simulink model "model"  (R2023b)
settings: Solver=VariableStepAuto  StartTime=0  StopTime=simtime  FixedStep=0.001  RelTol=1e-3
values from neighbouring files (symbols this model uses):
  A = 93.086154    [project1.m]
  Af = 2.2    [project1.m]
  B = 2.5373490    (= 2.537349)    [project1.m]
  C = 0.38382359    [project1.m]
  Cd = 0.3    [project1.m]
  Crr = 0.015    [project1.m]
  D = 0    [project1.m]
  g0 = 3.173    [project1.m]
  I = 0.1    [project1.m]
  M = 1200    [project1.m]
  P = 10    [project1.m]
  Rw = 0.281154    [project1.m]
libraries: autolibshared x1
settings Model: Creator=qwert  LastModifiedBy=chall2022

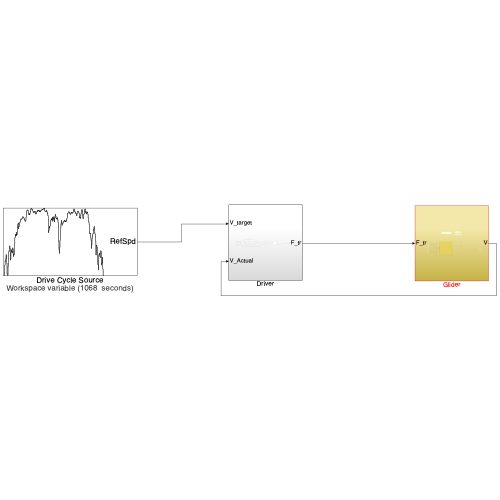
[thumbnail: Simulink's stored preview of the top-level diagram]
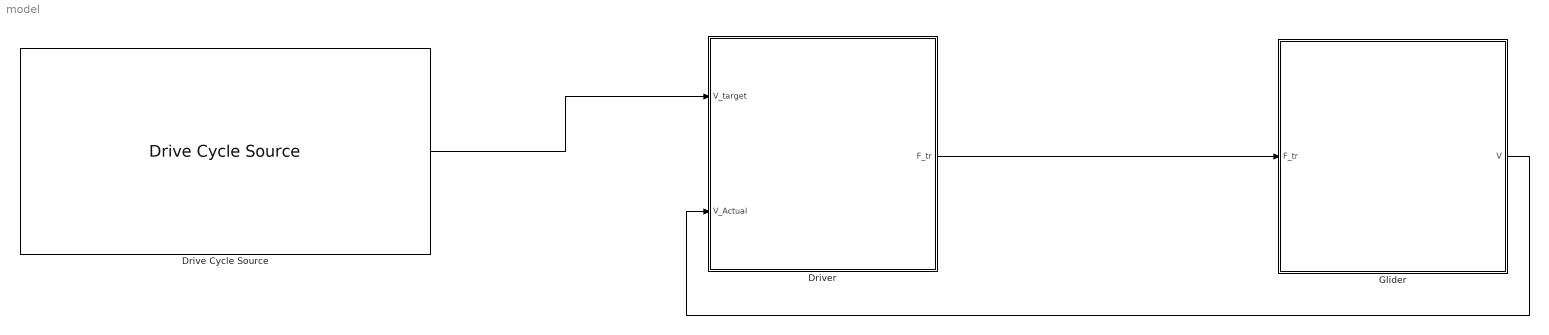
== system model ==
  Drive Cycle Source : autolibshared/Drive Cycle Source  cycleVar=Workspace variable  wsVar=Drivecycle  fileVar=cycleFTP75.mat  tfinal="1068  seconds"  cycleRepeat=off  outAccPort=off  outGearPort=off  gearList=No gear data  t_wot1=5  xdot_woto=0  xdot_wot1=30  t_wot2=20  xdot_wot2=0  t_wotend=30  srcUnit=m/s  outUnit=m/s  srcAccUnit=m/s/s  outAccUnit=m/s^2  dt=0  aMode=1  faultOption=off  velBnd=2  velBndUnit=mph  inUnit=m/s  timeBnd=1  failOption=off  stopSim=off  maxFaultCnt=10  maxFaultTime=2  maxTotFaultTime=15  traceOption=off  dtTrace=1  traceWindow=10  lastDCname=Custom Data Set  lastOutUnit=mph  lastDT=0  lastTB=1  lastSB=2  forceCalcBound=off
  Driver : Subsystem
  Glider : Subsystem
  wires:
  Driver/1(F_tr) -> Glider/1(F_tr)
  Drive Cycle Source/1 -> Driver/1(V_target)
  Glider/1(V) -> Driver/2(V_Actual)

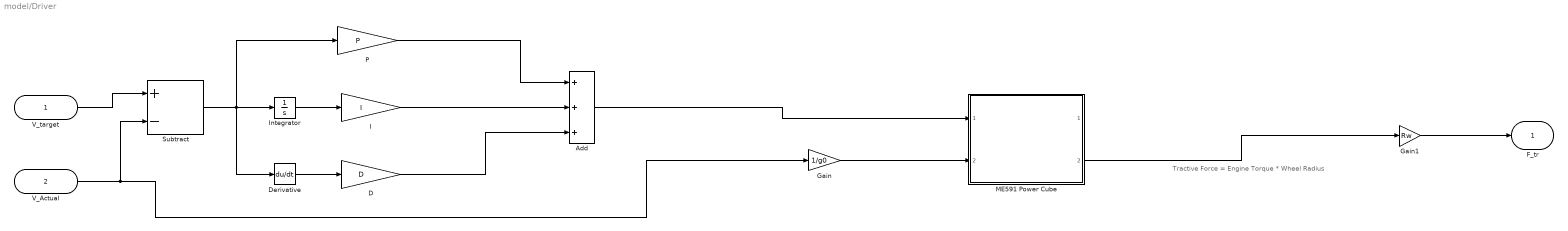
== system model/Driver ==
  note: Tractive Force = Engine Torque * Wheel Radius
  V_target : Inport
  V_Actual : Inport  Port=2
  Add : Sum  Inputs=+++
  D : Gain  Gain=D
  Derivative : Derivative
  Gain : Gain  Gain=1/g0
  Gain1 : Gain  Gain=Rw
  I : Gain  Gain=I
  Integrator : Integrator
  ME591 Power Cube : Subsystem  ReferencedSubsystem=ME591_Power_Cube
  P : Gain  Gain=P
  Subtract : Sum  Inputs=+-
  F_tr : Outport
  wires:
  I/1 -> Add/2
  P/1 -> Add/1
  D/1 -> Add/3
  Derivative/1 -> D/1
  Integrator/1 -> I/1
  V_Actual/1 -> Subtract/2, Gain/1
  Gain/1 -> ME591 Power Cube/2
  Gain1/1 -> F_tr/1
  Add/1 -> ME591 Power Cube/1
  V_target/1 -> Subtract/1
  Subtract/1 -> Derivative/1, P/1, Integrator/1
  ME591 Power Cube/2 -> Gain1/1

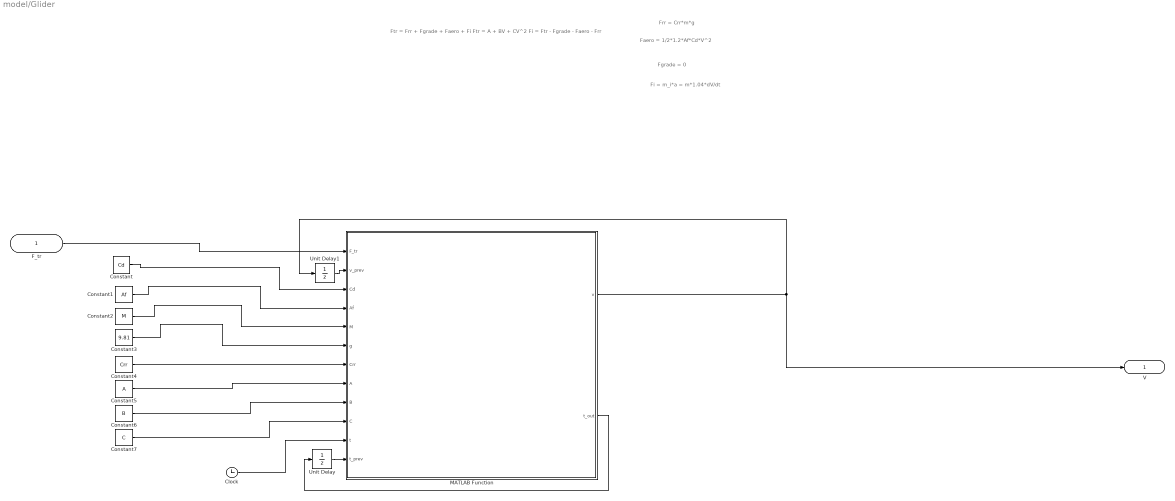
== system model/Glider ==
  note: Fi = m_i*a = m*1.04*dV/dt
  note: Faero = 1/2*1.2*Af*Cd*V^2
  note: Frr = Crr*m*g
  note: Ftr = Frr + Fgrade + Faero + Fi
      | Ftr = A + BV + CV^2
      | Fi = Ftr - Fgrade - Faero - Frr
  note: Fgrade = 0
  F_tr : Inport
  Clock : Clock
  Constant : Constant  Value=Cd
  Constant1 : Constant  Value=Af
  Constant2 : Constant  Value=M
  Constant3 : Constant  Value=9.81
  Constant4 : Constant  Value=Crr
  Constant5 : Constant  Value=A
  Constant6 : Constant  Value=B
  Constant7 : Constant  Value=C
  MATLAB Function : MATLAB Function  TreatAsAtomicUnit=on
  Unit Delay : UnitDelay  SampleTime=-1  HasFrameUpgradeWarning=on
  Unit Delay1 : UnitDelay  SampleTime=-1  HasFrameUpgradeWarning=on
  V : Outport
  wires:
  F_tr/1 -> MATLAB Function/1(F_tr)
  MATLAB Function/1(v) -> Unit Delay1/1, V/1
  Constant/1 -> MATLAB Function/3(Cd)
  Constant1/1 -> MATLAB Function/4(Af)
  Constant2/1 -> MATLAB Function/5(M)
  Constant3/1 -> MATLAB Function/6(g)
  Constant4/1 -> MATLAB Function/7(Crr)
  Constant5/1 -> MATLAB Function/8(A)
  Constant6/1 -> MATLAB Function/9(B)
  Constant7/1 -> MATLAB Function/10(C)
  MATLAB Function/2(t_out) -> Unit Delay/1
  Clock/1 -> MATLAB Function/11(t)
  Unit Delay/1 -> MATLAB Function/12(t_prev)
  Unit Delay1/1 -> MATLAB Function/2(v_prev)

== matlab function model/Glider/MATLAB Function ==
  data: F_tr input; v output; v_prev input; Cd input; Af input; M input; g input; Crr input; A input; B input; C input; t input; t_prev input; t_out output
function [v, t_out]= fcn(F_tr, v_prev, Cd, Af, M, g, Crr, A, B, C, t, t_prev)

    v = 0;

    dt = t - t_prev;
    t_out = t;
    
    %% Calculate resistive forces
    % Aerodynamic drag
    F_drag = 0.5 * 1.2 * Cd * Af * v_prev^2;
    
    % Rolling resistance
    F_rolling = Crr * M * g;
    
    % Coasting down equation (A + B*v + C*v^2)
    F_coast = A + B * v_prev + C * v_prev^2;

    %% Net force acting on the vehicle
    F_net = F_tr - (F_drag + F_rolling + F_coast);

    %% Acceleration of the vehicle
    a = F_net / M;

    %% Update the velocity using basic kinematics
    v = v_prev + a * dt; % New velocity (m/s)
    
    % Ensure that velocity does not become negative
    if v < 0
        v = 0;
    end

end
